simulink model "flightControlSystem"  (R2024b)
settings: Solver=ode3  StartTime=0  StopTime=TFinal  FixedStep=Ts  RelTol=1e-3  EnableMultiTasking=on
undefined symbols (not defined in the file): codertarget, Controller, DiscIntNeverNeededParam, Discrete, Estimator, g, gray, init, orient_ref, pos_ref, Rec, SDTV, Sensors, strel, Time, Ts, var_acc_angle_N, var_bias_gyr_N, var_gyro_p_N, Vehicle
libraries: simulink x45, slpidlib x4, ctrlSharedLib x4, sharedtransform x3, visionstatistics x2, visionconversions x2, visionmorphops x2, visiontextngfix x2, parrotlib x1
(part 3 of 3)

== matlab function flightControlSystem/Image Processing System/Linia na Punkty ==
  data: out output; binaryImage input; pts_vector output; pts output; out_2 output; out_3 output; out_4 output
function [out, pts_vector, pts, out_2, out_3, out_4] = ZnajdzPunkty(binaryImage)
    %% 1. JAWNA DEKLARACJA ROZMIARÓW
    MAX_VECTOR_LEN = 20; 
    MAX_PAIRS      = 10; 
    TARGET_COUNT   = 3;  
    
    persistent prev_pts prev_count
    
    if isempty(prev_pts)
        prev_pts = zeros(MAX_PAIRS, 2, 'single');
        prev_count = 0;
    end
    
    pts = zeros(MAX_PAIRS, 2, 'single');        
    pts_vector = zeros(1, MAX_VECTOR_LEN, 'single'); 
    
    %% 2. Przetwarzanie Obrazu
    skel_base = bwmorph(binaryImage, 'skel', Inf);
    points_cloud_img = bwmorph(skel_base, 'branchpoints'); 
    
    %% 3. Pobranie chmury punktów
    [y_all, x_all] = find(points_cloud_img);
    num_pixels = numel(x_all);
    
    % PLAN AWARYJNY: Jeśli branchpoints nic nie zwrócił
    if num_pixels < 2
        endpoints_img = bwmorph(skel_base, 'endpoints');
        [y_all, x_all] = find(endpoints_img);
        num_pixels = numel(x_all);
    end

    x_s = single(x_all);
    y_s = single(y_all);
    
    %% 4. ALGORYTM GEOMETRYCZNY (Regresja)
    selected_pts = zeros(TARGET_COUNT, 2, 'single');
    sel_count = 0;
    
    % Parametry
    MIN_LINE_LEN_SQ = single(400.0); % (20px)^2
    CORNER_THRESH   = single(10.0);  % Próg błędu
    MIN_SEGMENT_SQ  = single(400.0); % (20px)^2 - min odległość rogu od końców
    
    if num_pixels >= 2
        % KROK 1: Start (Dół)
        [~, idx_start] = max(y_s);
        P_start = [x_s(idx_start), y_s(idx_start)];
        
        % KROK 2: Koniec (Max dystans)
        max_dist_sq = single(-1);
        idx_end = -1;
        
        for k = 1:num_pixels
            d_sq = (x_s(k) - P_start(1))^2 + (y_s(k) - P_start(2))^2;
            if d_sq > max_dist_sq
                max_dist_sq = d_sq;
                idx_end = k;
            end
        end
        
        if max_dist_sq > MIN_LINE_LEN_SQ
            P_end = [x_s(idx_end), y_s(idx_end)];
            
            % KROK 3: Szukaj ROGU
            max_deviation = single(-1);
            idx_corner = -1;
            
            vx = P_end(1) - P_start(1);
            vy = P_end(2) - P_start(2);
            len_line = sqrt(vx*vx + vy*vy) + 0.001;
            
            for k = 1:num_pixels
                px = x_s(k); py = y_s(k);
                cross_prod = abs(vx*(P_start(2) - py) - (P_start(1) - px)*vy);
                dist_to_line = cross_prod / len_line;
                
                if dist_to_line > max_deviation
                    max_deviation = dist_to_line;
                    idx_corner = k;
                end
            end
            
            % --- KROK 4: Decyzja ---
            sel_count = 3; 
            selected_pts(1, :) = P_start;
            
            is_valid_corner = false;
            % FIX: Jawna inicjalizacja jako single!
            P_corner = single([0 0]); 
            
            if max_deviation > CORNER_THRESH
                P_cand = [x_s(idx_corner), y_s(idx_corner)];
                
                d_start = (P_cand(1)-P_start(1))^2 + (P_cand(2)-P_start(2))^2;
                d_end   = (P_cand(1)-P_end(1))^2   + (P_cand(2)-P_end(2))^2;
                
                if d_start > MIN_SEGMENT_SQ && d_end > MIN_SEGMENT_SQ
                    is_valid_corner = true;
                    P_corner = P_cand;
                end
            end
            
            if is_valid_corner
                selected_pts(2, :) = P_corner;
                selected_pts(3, :) = P_end;
            else
                P_mid = (P_start + P_end) * 0.5;
                selected_pts(2, :) = P_mid;
                selected_pts(3, :) = P_end;
            end
        else
            % Za krótka linia
            sel_count = 3;
            selected_pts(1,:) = P_start;
            selected_pts(2,:) = P_start;
            selected_pts(3,:) = P_start;
        end
    end
    
    %% 5. STABILIZACJA I SORTOWANIE
    
    if sel_count == 3
        if selected_pts(1, 2) < selected_pts(3, 2)
            swap_pts = selected_pts;
            selected_pts(1,:) = swap_pts(3,:);
            selected_pts(3,:) = swap_pts(1,:);
        end
    end
    
    if sel_count > 0 && prev_count > 0
        ALPHA = single(0.7);
        for k = 1:sel_count
            min_d = single(900.0);
            best_idx = -1;
            for p = 1:min(prev_count, MAX_PAIRS) 
                 if p <= 3 
                    dx = selected_pts(k,1) - prev_pts(p,1);
                    dy = selected_pts(k,2) - prev_pts(p,2);
                    dd = dx*dx + dy*dy;
                    if dd < min_d
                        min_d = dd;
                        best_idx = p;
                    end
                 end
            end
            if best_idx ~= -1
                selected_pts(k, 1) = ALPHA*selected_pts(k,1) + (1-ALPHA)*prev_pts(best_idx,1);
                selected_pts(k, 2) = ALPHA*selected_pts(k,2) + (1-ALPHA)*prev_pts(best_idx,2);
            end
        end
    end

    % --- FIX WYMIARÓW ---
    pts = zeros(MAX_PAIRS, 2, 'single');
    for k = 1:sel_count
        pts(k, :) = selected_pts(k, :);
    end
    
    prev_pts = pts;
    prev_count = sel_count;
    
    %% 6. Wyjścia
    for k = 1:sel_count
        pts_vector(2*k - 1) = pts(k, 1);
        pts_vector(2*k)     = pts(k, 2);
    end
    
    %% 7. Debug
    out = binaryImage;
    out_2 = points_cloud_img; 
    out_4 = false(size(binaryImage)); 
    out_3 = false(size(binaryImage)); 
    [rows_img, cols_img] = size(binaryImage);
    
    for k = 1:sel_count
        c = round(pts(k, 1));
        r = round(pts(k, 2));
        if c >= 1 && c <= cols_img && r >= 1 && r <= rows_img
            out_3(r, c) = true;
            if c > 1 && c < cols_img && r > 1 && r < rows_img
                out_3(r-1, c) = true; out_3(r+1, c) = true;
                out_3(r, c-1) = true; out_3(r, c+1) = true;
            end
        end
    end
end

== matlab function flightControlSystem/Control System/Controller/Position Controller/Position error transformation (Earth to Body frame) ==
  data: yaw input; xy_err_earth input; xy_err_body output
function xy_err_body = fcn(yaw,xy_err_earth)

transformation = [cos(yaw), sin(yaw); -sin(yaw),  cos(yaw)];
xy_err_body = transformation * xy_err_earth;


end

== stateflow chart flightControlSystem/Control System/Path Planning/Algorytm lotu ==
  state Hover
    entry:
    %
    xout = 0;
    yout = 0;
    zout = -1;
    %
    yawout = 0;
    pitchout = 0;
    rollout = 0;
  state InfLoop
    state FindTheLine
      entry:
      % Inicjalizacja wyjść na start
      xout = xestim;
      yout = yestim;
      zout = zestim;
      C = [80, 60];
      % Parametry regulatora
      K_P = 0.00001;
      MAX_SPEED = 0.005;   % Limit prędkości
      tol = 5;
      DESC = 0;
      during:
      % 1. Pobierz punkt odniesienia
      TargetPoint = Coordinates(2, :);
      % 2. Oblicz błąd
      err_body_forward = (C(2) - TargetPoint(2)); % Błąd w osi Przód-Tył
      err_body_side    = (C(1) - TargetPoint(1)); % Błąd w osi Lewo-Prawo
      % 3. Oblicz prędkości w układzie DRONA
      v_fwd = err_body_forward * K_P;
      v_side = -err_body_side * K_P; % Minus, bo oś jest odwrócona
      % Ograniczenie prędkości
      v_fwd  = max(min(v_fwd, MAX_SPEED), -MAX_SPEED);
      v_side = max(min(v_side, MAX_SPEED), -MAX_SPEED);
      if abs(err_body_forward) <= tol
      v_fwd = 0;
      end
      if abs(err_body_side) <= tol
      v_side = 0;
      end
      % 5. Transformacja na układ GLOBALNY
      yaw = ayaw; % Pobierz aktualny kąt w radianach
      vx_global = v_fwd * cos(yaw) - v_side * sin(yaw);
      vy_global = v_fwd * sin(yaw) + v_side * cos(yaw);
      % 6. Ruch
      xout = xout + vx_global;
      yout = yout + vy_global;
      zout = -1;
    state FindTheState
      entry:
      % --- 1. POBRANIE DANYCH ---
      P1 = Coordinates(1, :);
      P2 = Coordinates(2, :);
      P3 = Coordinates(3, :);
      Land_Flag   = Coordinates(4, 1); % 1 jeśli wykryto strefę lądowania
      Land_Target = Coordinates(5, :); % [X, Y] lądowiska
      C  = [80, 60];
      % Tolerancje
      pos_tol = 5;    % Tolerancja pozycji
      an_tol = 5;     % Tolerancja kąta
      % --- 2. RESET FLAG ---
      STATE = 0;
      ROTATE = 0;
      BLANK  = 0;
      START  = 0;
      TURN_POINT = 0;
      GOSTRAIGHT = 0;
      LANDING = 0;
      % Domyślny cel
      TARGET_POINT = P2;
      error_y = 0;
      %% --- 3. LOGIKA ---
      % A. CZY WYKRYTO LĄDOWISKO? (PRIORYTET 1)
      if Land_Flag == 1
      STATE = 9;       % Stan 9 = Lądowanie
      LANDING = 1;
      TARGET_POINT = Land_Target;
      error_y = C(2) - TARGET_POINT(2);
      else
      % --- STARA LOGIKA ŚLEDZENIA LINII (PRIORYTET 2) ---
      % B. CZY WYKRYTO PUNKTY?
      if isequal(P1, [0 0]) && isequal(P2, [0 0]) && isequal(P3, [0 0])
      BLANK = 1;
      STATE = 1;
      else
      % C. CZY DRON NAD LINIĄ?
      check_C1 = abs(Center1(1) - C(1)) <= pos_tol;
      check_C2 = false;
      if ~isequal(P3, [0 0])
      check_C2 = abs(Center2(1) - C(1)) <= pos_tol;
      end
      if ~(check_C1 || check_C2)
      % Dron obok linii -> FindTheLine
      STATE = 2;
      START = 0;
      else
      % Dron nad linią
      START = 1;
      % --- D. ANALIZA WZDŁUŻNA (Y) ---
      is_at_or_past_target = TARGET_POINT(2) >= (C(2) - pos_tol);
      if is_at_or_past_target
      % === STREFA ZA P2  ===
      % Jeśli błąd kąta -> obrót
      if ~isequal(P3, [0 0]) && abs(Alpha2) >= an_tol
      STATE = 3;
      TURN_POINT = 1;
      else
      STATE = 4;
      if ~isequal(P3, [0 0])
      TARGET_POINT = P3;
      else
      TARGET_POINT = P2;
      end
      GOSTRAIGHT = 1;
      end
      else
      % === STREFA PRZED P2 ===
      % Jeśli błąd kąta -> obrót
      if abs(Alpha1) >= an_tol % && abs(Alpha2) <= 2*an_tol
      STATE = 5;
      ROTATE = 1;
      else
      STATE = 7;
      TARGET_POINT = P2;
      GOSTRAIGHT = 1;
      end
      end
      % Blad do lotu prosto
      error_y = C(2) - TARGET_POINT(2);
      end
      end
      end
      angle = rad2deg(ayaw);
    state GOSTRAIGHT
      entry:
      % Parametry regulatora
      K_P = 0.00001;
      MAX_SPEED = 0.005;   % Limit prędkości
      during:
      cmd_speed = K_P * error_y;
      % Ograniczenie prędkości
      if cmd_speed > MAX_SPEED
      speed = MAX_SPEED;
      elseif cmd_speed < -MAX_SPEED
      speed = -MAX_SPEED;
      else
      speed = cmd_speed;
      end
      % WYKONANIE RUCHU
      xout = xout + speed * cos(ayaw);
      yout = yout + speed * sin(ayaw);
      zout = -1;     % Stała wysokość
    state WAIT1
      entry:
      %
      xout = xestim;
      yout = yestim;
      zout = -1;
      %
    state ROTATE
      entry:
      xout = xestim; %
      yout = yestim; %i
      zout = zestim;
      yawout = ayaw;
      an_tol = 3;
      END = 0;
      during:
      if Alpha1 < -an_tol
      yawout = yawout + 0.001;
      END = 0;
      elseif Alpha1 > an_tol
      yawout = yawout - 0.001;
      END = 0;
      else
      % Dron w strefie tolerancji -> Koniec obracania
      END = 1;
      ROTATE = 0;
      end
    state WAIT2
      entry:
      %
      xout = xestim;
      yout = yestim;
      zout = -1;
      %
    state CENTER
      entry:
      % Inicjalizacja wyjść na start
      xout = xestim;
      yout = yestim;
      zout = zestim;
      C = [80, 60];
      % Parametry regulatora
      K_P = 0.00001;
      MAX_SPEED = 0.005;   % Limit prędkości
      tol = 5;
      DESC = 0;
      during:
      % 1. Pobierz punkt odniesienia
      TargetPoint = Coordinates(5, :);
      % 2. Oblicz błąd
      err_body_forward = (C(2) - TargetPoint(2)); % Błąd w osi Przód-Tył
      err_body_side    = (C(1) - TargetPoint(1)); % Błąd w osi Lewo-Prawo
      % 3. Oblicz prędkości w układzie DRONA
      v_fwd = err_body_forward * K_P;
      v_side = -err_body_side * K_P; % Minus, bo oś jest odwrócona
      % Ograniczenie prędkości
      v_fwd  = max(min(v_fwd, MAX_SPEED), -MAX_SPEED);
      v_side = max(min(v_side, MAX_SPEED), -MAX_SPEED);
      if abs(err_body_forward) <= tol
      v_fwd = 0;
      end
      if abs(err_body_side) <= tol
      v_side = 0;
      end
      % 5. Transformacja na układ GLOBALNY
      yaw = ayaw; % Pobierz aktualny kąt w radianach
      vx_global = v_fwd * cos(yaw) - v_side * sin(yaw);
      vy_global = v_fwd * sin(yaw) + v_side * cos(yaw);
      % 6. Ruch
      xout = xout + vx_global;
      yout = yout + vy_global;
      zout = -1;
      if abs(err_body_forward) <= tol && abs(err_body_side) <= tol
      DESC = 1;
      else
      DESC = 0;
      end
    state WAIT3
      entry:
      %
      xout = xestim;
      yout = yestim;
      zout = -1;
      %
    state LAND
      zout = zout + 0.001;
      if zout < 0.1
      zout = 0;
      end
    state TURN_POINT
      entry:
      xout = xestim; %
      yout = yestim; %
      zout = zestim;
      yawout = ayaw;
      an_tol = 3;
      END = 0;
      during:
      if Alpha2 < -an_tol
      yawout = yawout + 0.001;
      END = 0;
      elseif Alpha2 > an_tol
      yawout = yawout - 0.001;
      END = 0;
      else
      % Dron w strefie tolerancji -> Koniec obracania
      END = 1;
      TURN_POINT = 0;
      end
    (default) -> FindTheState
    FindTheState -> FindTheLine [order 3] : [START==0 && LANDING == 0]
    GOSTRAIGHT -> FindTheState : [after(return_time,sec)]
    FindTheState -> GOSTRAIGHT [order 4] : [GOSTRAIGHT == 1]
    FindTheLine -> FindTheState : [ after(return_time,sec)]
    FindTheState -> WAIT1 [order 1] : [ROTATE==1]
    WAIT1 -> ROTATE : [after(1,sec)]
    ROTATE -> FindTheState : [END == 1&&after(1,sec)]
    FindTheState -> WAIT2 [order 2] : [LANDING == 1]
    WAIT2 -> CENTER : [after(5,sec)]
    FindTheState -> WAIT3 [order 5] : [TURN_POINT==1]
    WAIT3 -> state195 : [after(return_time,sec)]
    CENTER -> LAND : [DESC == 1]
    state195 -> FindTheState : [END == 1&&after(1,sec)]
  (default) -> Hover
  Hover -> InfLoop : [after(5,sec)]
  data: Alpha1 input; Alpha2 input; Center1 input; Center2 input; ayaw input single; apitch input single; aroll input single; xestim input single; yestim input single; zestim input single; xout output single; yout output single; zout output single; yawout output single; pitchout output single; rollout output; tolerance local single; speed local single; C local single; Coordinates input single; tol local; BLANK local; P1 output single; P2 output single; P3 output; ROTATE local single; END local single; an_tol local single; TARGET_POINT local single; K_P local single; MAX_SPEED local single; cmd_speed local; angle output; TURN_POINT local; target local; an_tol_rad local; current_yaw local; error local; step local; target_yaw local; turn_angle_rad local; err_img_y local single; err_img_x local single; vy local single; vx local single; line_center_y local; line_center_x local; AB local; BC local; AC local; segment_center_x local; ROTATE_FLAG local; NEXT_ROTATE local; pos_tol local; tol_pos local; tol_x local; tol_y local; Target local; T_tol local; v_fwd local single; v_side local single; yaw local; vy_global local single; err_body_forward local; vx_global local single; TargetPoint local; err_body_side local; error_y local single; STATE output; is_at_or_past_P2 local; on_line_1 local; on_line_2 local; check_C1 local; check_C2 local; DESCENT_SPEED local; MAX_SPEED_XY local single; ALIGN_TOL local; LAND_ALT_LIMIT local; Has_Visual local; is_centered local; Land_Target local; LANDING local; K_P_XY local; Land_Flag output; START local; GOSTRAIGHT local; check_C3 local; dist1 local; dist3 local; dist2 local; min_dist local; check_C4 local; is_at_or_past_target local; DESC local; return_time local =0.8

== matlab function flightControlSystem/Control System/Path Planning/Znajdź kąty ==
  data: Coordinates input single; A1 output single; Alpha1 output single; Center1 output single; A2 output single; Alpha2 output single; Center2 output; Coordinates output
function [A1,Alpha1,Center1,A2,Alpha2,Center2,Coordinates] = oblicz_katy(Coordinates)
%% 
% Camera_center = [60, 80]; % Camera center[y,x]: y=60 (0 at top), x=80 (0 at the left)
% Pobierz punkty
P1 = Coordinates(1, :);
P2 = Coordinates(2, :);
P3 = Coordinates(3, :);

%% Oblicz parametry
% Linia 1
A1 = (P2(1)-P1(1))/(P2(2)-P1(2));
Alpha1 = rad2deg(atan(A1));  % kąt w stopniach
Center1 = [(P2(1)+P1(1))*0.5, (P2(2)+P1(2))*0.5]; % środek linii

% Linia 2
A2 = (P3(1)-P2(1))/(P3(2)-P2(2)); 
Alpha2 = rad2deg(atan(A2)); % kąt w stopniach
Center2 = [(P3(1)+P2(1))*0.5, (P3(2)+P2(2))*0.5]; % środek linii

== matlab function flightControlSystem/Image Processing System/MATLAB Function ==
  data: Area input; Centroid input; Eccentricity input; MajorAxis input; MinorAxis input; pts_in input; pts_out output
function pts_out = WykryjLadowisko(Area, Centroid, Eccentricity, MajorAxis, MinorAxis, pts_in)
    
    % --- KONFIGURACJA ---
    MIN_AREA = single(500);       
    MAX_ECCENTRICITY = single(0.95); 
    AREA_TOLERANCE = single(0.2); 
    
    % Przepisujemy wejście na wyjście (kopiujemy linię)
    pts_out = pts_in;
    
    % INICJALIZACJA LĄDOWISKA (Resetujemy punkty 4 i 5)
    % Punkt 4: Flaga [CzyWykryto, 0]
    % Punkt 5: Cel   [X, Y]
    pts_out(4, :) = single([0, 0]); 
    pts_out(5, :) = single([0, 0]);
    
    % Szukamy najlepszego kandydata
    num_blobs = numel(Area);
    best_score = single(0);
    
    for k = 1:num_blobs
        % 1. Filtr Wielkości
        current_area = single(Area(k)); 
        
        if current_area > MIN_AREA
            
            % 2. Filtr Kształtu (Mimośród)
            if Eccentricity(k) < MAX_ECCENTRICITY
                
                % 3. Filtr Matematyczny (Czy to elipsa?)
                radius_major = MajorAxis(k) / 2.0;
                radius_minor = MinorAxis(k) / 2.0;
                theoretical_area = single(pi) * radius_major * radius_minor;
                
                ratio = abs(current_area - theoretical_area) / theoretical_area;
                
                if ratio < AREA_TOLERANCE
                    % To jest nasze lądowisko!
                    
                    if current_area > best_score
                        best_score = current_area; 
                        
                        % --- ZAPIS DO MACIERZY PTS ---
                        
                        % Punkt 4: Flaga wykrycia (1 w pierwszej kolumnie)
                        pts_out(4, 1) = single(1); 
                        pts_out(4, 2) = single(0); % Druga kolumna nieużywana
                        
                        % Punkt 5: Współrzędne celu [X, Y]
                        pts_out(5, 1) = single(Centroid(k, 1)); % X
                        pts_out(5, 2) = single(Centroid(k, 2)); % Y
                    end
                end
            end
        end
    end
end

== matlab function flightControlSystem/Image Processing System/Analiza jakościowa/Analiza_bledu ==
  data: thin_out output; dist_error output; dist_error_tol output; is_perfect_center output; binaryImage input; isCircleDetected input
function [thin_out, dist_error, dist_error_tol, is_perfect_center] = AnalizaThin(binaryImage, isCircleDetected)
    % --- KONFIGURACJA ---
    C_X = single(80);
    C_Y = single(60);
    TOLERANCE = single(5.0); % Tolerancja w pikselach
    
    % --- 1. PRE-PROCESSING ---
    img_clean = bwmorph(binaryImage, 'clean');
    
    % --- 2. OPERACJA THIN ---
    line_raw = bwmorph(img_clean, 'thin', Inf);
    
    % --- 3. POST-PROCESSING ---
    line_thin = bwmorph(line_raw, 'spur', 7);
    line_thin = bwmorph(line_thin, 'clean');
    
    % Wyjście obrazu
    thin_out = line_thin; 
    
    % Inicjalizacja zmiennych wyjściowych
    dist_error = single(0);
    dist_error_tol = single(0); % Domyślnie 0 (w strefie tolerancji)
    is_perfect_center = single(0);

    % --- 4. PRIORYTET: CZY WYKRYTO LĄDOWISKO (KOŁO)? ---
    if isCircleDetected == 1
        % Ignorujemy błąd linii, zwracamy zera (zainicjowane wyżej)
        return; 
    end

    % --- 5. CZY JESTEŚMY IDEALNIE NA LINII? ---
    if line_thin(60, 80)
        is_perfect_center = single(1);
        % Błędy są 0, return wychodzi z funkcji
        return; 
    end
    
    % --- 6. OBLICZANIE ODLEGŁOŚCI ---
    [y_pts, x_pts] = find(line_thin);
    
    if isempty(x_pts)
        % Nie ma linii -> Błąd maksymalny
        raw_error = single(100);
    else
        min_dist_sq = single(1000000);
        num_pts = numel(x_pts);
        
        for k = 1:num_pts
            dx = single(x_pts(k)) - C_X;
            dy = single(y_pts(k)) - C_Y;
            d_sq = dx*dx + dy*dy;
            
            if d_sq < min_dist_sq
                min_dist_sq = d_sq;
            end
        end
        
        raw_error = sqrt(min_dist_sq);
    end
    
    % Przypisanie błędu surowego
    dist_error = raw_error;
    
    % --- 7. APLIKACJA TOLERANCJI (Strefa Martwa) ---
    if raw_error > TOLERANCE
        dist_error_tol = raw_error;
    else
        dist_error_tol = single(0);
    end
end

== matlab function flightControlSystem/Image Processing System/Analiza jakościowa/Analiza/isCircle ==
  data: eccentricity input; isCircleDetected output; centroid input; circle_x output; circle_y output
function [isCircleDetected,circle_x,circle_y] = isCircle(eccentricity,centroid)

isCircleDetected = 0;

mid_coords = [80,60];

circle_x = 0;
circle_y = 0;

for idx = 1:3
    if(eccentricity(idx)<0.2 && eccentricity(idx)>0)
        isCircleDetected = 1;
        if isCircleDetected == 1
           n = idx;
           circle_x = centroid(n,1) - mid_coords(1);
           circle_y = centroid(n,2) - mid_coords(2);
        end
    end
end

== matlab function flightControlSystem/Image Processing System/Analiza jakościowa/Analiza/isCircle1 ==
  data: eccentricity input; centroid input; track_x output; track_y output
function [track_x,track_y] = notCircle(eccentricity,centroid)

mid_coords = [80,60];

track_x = 0;
track_y = 0;

for idx = 1:3
    if(eccentricity(idx)>0.2)
        n = idx;
        track_x = centroid(n,1) - mid_coords(1);
        track_y = centroid(n,2) - mid_coords(2);
    end
end
